simulink library "periodicControllerExp_wCtrlAllocation"  (R2020a)
settings: Solver=VariableStepAuto  StartTime=0.0  StopTime=10.0  RelTol=1e-3
undefined symbols (not defined in the file or in its folder): FLIGHTCONTROLLER, rollAmp, rollFreq, rollKD, rollKP, startControl, tow_speed, vhcl, yawAmp, yawFreq, yawKP
libraries: hiToLoElevationControllerExp x1, ctrlAllocMatrix_cl x1, filteredPIDController_ul x1
settings Model: Creator=jcreed2  LastModifiedBy=jcreed2

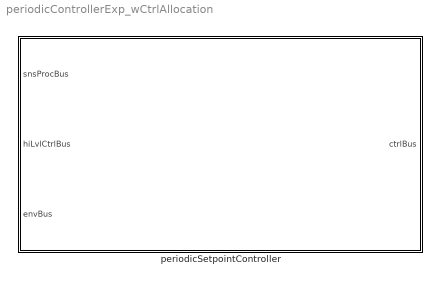
== system periodicControllerExp_wCtrlAllocation ==
  periodicSetpointController : Subsystem  VariantControl=strcmpi(FLIGHTCONTROLLER,'periodicSetpointController')

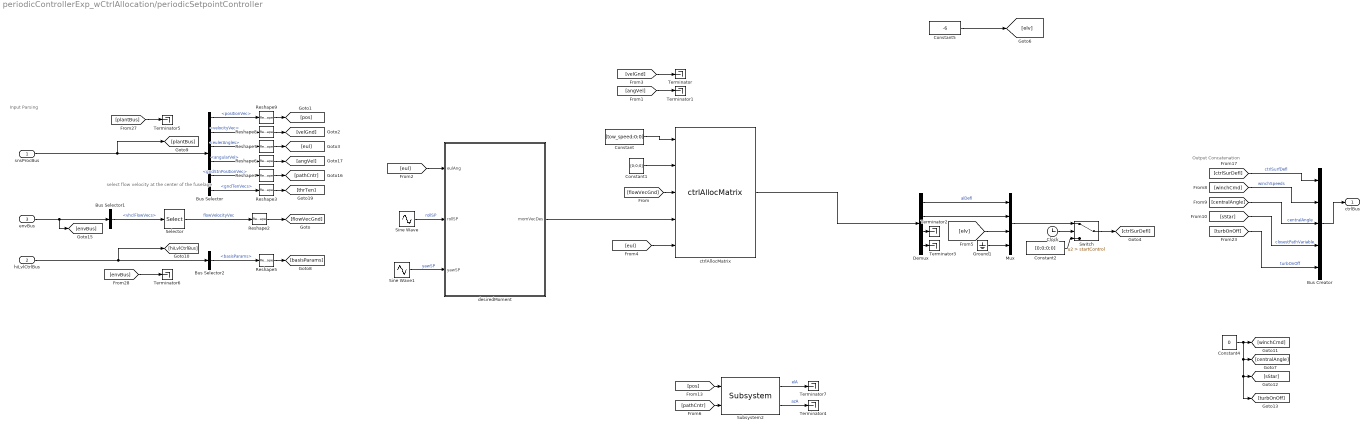
== system periodicControllerExp_wCtrlAllocation/periodicSetpointController ==
  note: select flow velocity at the center of the fuselage
  note: Input Parsing
  note: Output Concatenation
  snsProcBus : Inport  OutDataTypeStr=Bus: sensorsProcessingBus
  hiLvlCtrlBus : Inport  Port=2  OutDataTypeStr=Bus: hiLvlCtrlBus
  envBus : Inport  Port=3  OutDataTypeStr=Bus: envBus
  Bus Creator : BusCreator  Inputs=5  OutDataTypeStr=Bus: fltCtrlBus
      settings: InheritFromInputs=off
  Bus Selector : BusSelector  OutputSignals=positionVec,velocityVec,eulerAngles,angularVel,gndStnPositionVec,gndTenVecs
  Bus Selector1 : BusSelector  OutputSignals=vhclFlowVecs
  Bus Selector2 : BusSelector  OutputSignals=basisParams
  Clock : Clock
  Constant : Constant  Value=[tow_speed;0;0]
  Constant1 : Constant  Value=[0;0;0]
  Constant2 : Constant  Value=[0;0;0;0]
  Constant4 : Constant  Value=0
  Constant5 : Constant  Value=-6
  Demux : Demux
  Ground1 : Ground
  Mux : Mux
  Reshape{1..3,5..9} (8 alike) : Reshape  OutputDimensionality=Column vector (2-D)
  Selector : Selector  NumberOfDimensions=2  InputPortWidth=3  IndexOptions=Select all,Index vector (dialog)  Indices=[1 3],5  OutputSizes=1,1
  Sine Wave : Sin  Amplitude=rollAmp  Bias=180  Frequency=rollFreq  SampleTime=0
  Sine Wave1 : Sin  Amplitude=yawAmp  Bias=pi  Frequency=yawFreq  SampleTime=0
  Subsystem2 : hiToLoElevationControllerExp/hiToLoElevationControllerExp/Subsystem  SystemSampleTime=-1  Latency=0  AutoFrameSizeCalculation=off
  Switch : Switch  Criteria=u2 > Threshold  Threshold=startControl  ZeroCross=off
  Terminator{,1..7} (8 alike) : Terminator
  ctrlAllocMatrix : ctrlAllocMatrix_cl/ctrlAllocMatrix  aeroStruct=vhcl.struct('OCT.aeroSurf')  fluidDensity=1000
  desiredMoment : Subsystem  mask{rollKp=rollKP, rollKd=rollKD, rollTau=.02, yawKp=yawKP}
      mask prompts: rollKp "roll kp"; rollKd "roll kd"; rollTau "roll time constant"; yawKp "yaw kp"
  ctrlBus : Outport  OutDataTypeStr=Bus: fltCtrlBus  VectorParamsAs1DForOutWhenUnconnected=off
  wires:
  Sine Wave/1 -> desiredMoment/2(rollSP)  "rollSP"
  [velGnd] -> Terminator/1
  Sine Wave1/1 -> desiredMoment/3(yawSP)  "yawSP"
  [eul] -> ctrlAllocMatrix/5
  [angVel] -> Terminator1/1
  [flowVecGnd] -> ctrlAllocMatrix/3
  [eul] -> desiredMoment/1(eulAng)
  Bus Selector/2 -> Reshape8/1  "<velocityVec>"
  Reshape3/1 -> [thrTen]
  Bus Selector/5 -> Reshape1/1  "<gndStnPositionVec>"
  Bus Selector/1 -> Reshape9/1  "<positionVec>"
  Reshape5/1 -> [basisParams]
  Reshape1/1 -> [pathCntr]
  envBus/1 -> [envBus], Bus Selector1/1
  snsProcBus/1 -> Bus Selector/1, [plantBus]
  hiLvlCtrlBus/1 -> [hiLvlCtrlBus], Bus Selector2/1
  Reshape2/1 -> [flowVecGnd]
  Bus Selector/4 -> Reshape6/1  "<angularVel>"
  Selector/1 -> Reshape2/1  "flowVelocityVec"
  Bus Selector2/1 -> Reshape5/1  "<basisParams>"
  Bus Selector/6 -> Reshape3/1  "<gndTenVecs>"
  [envBus] -> Terminator6/1
  Reshape6/1 -> [angVel]
  Reshape9/1 -> [pos]
  Bus Selector/3 -> Reshape7/1  "<eulerAngles>"
  Bus Selector1/1 -> Selector/1  "<vhclFlowVecs>"
  [plantBus] -> Terminator5/1
  Reshape7/1 -> [eul]
  Reshape8/1 -> [velGnd]
  [ctrlSurDefl] -> Bus Creator/1  "ctrlSurfDefl"
  [centralAngle] -> Bus Creator/3  "centralAngle"
  [turbOnOff] -> Bus Creator/5  "turbOnOff"
  [winchCmd] -> Bus Creator/2  "winchSpeeds"
  [sStar] -> Bus Creator/4  "closestPathVariable"
  Bus Creator/1 -> ctrlBus/1
  Constant4/1 -> [turbOnOff], [sStar], [centralAngle], [winchCmd]
  [elv] -> Mux/3
  desiredMoment/1(momVecDes) -> ctrlAllocMatrix/4
  Constant/1 -> ctrlAllocMatrix/1
  Constant1/1 -> ctrlAllocMatrix/2
  ctrlAllocMatrix/1 -> Demux/1
  Demux/1 -> Mux/1  "alDefl"
  Demux/2 -> Mux/2
  Ground1/1 -> Mux/4
  Constant5/1 -> [elv]
  Demux/3 -> Terminator2/1
  Demux/4 -> Terminator3/1
  Subsystem2/1 -> Terminator7/1  "elA"
  [pathCntr] -> Subsystem2/2
  [pos] -> Subsystem2/1
  Subsystem2/2 -> Terminator4/1  "azA"
  Clock/1 -> Switch/2
  Constant2/1 -> Switch/3
  Switch/1 -> [ctrlSurDefl]
  Mux/1 -> Switch/1

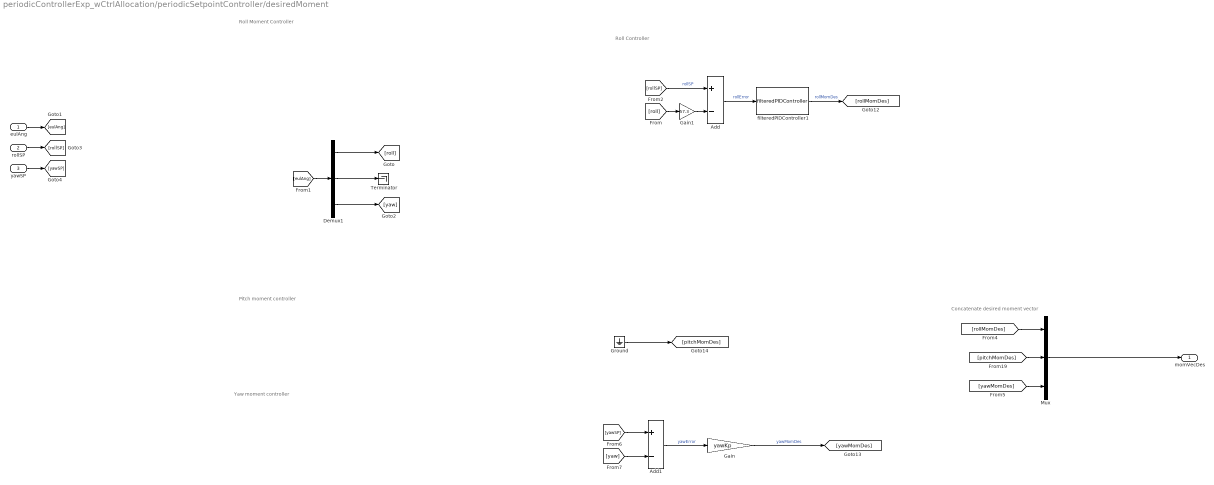
== system periodicControllerExp_wCtrlAllocation/periodicSetpointController/desiredMoment ==
  note: Pitch moment controller
  note: Roll Controller
  note: Yaw moment controller
  note: Roll Moment Controller
  note: Concatenate desired moment vector
  eulAng : Inport
  rollSP : Inport  Port=2
  yawSP : Inport  Port=3
  Add : Sum  Inputs=+-
  Add1 : Sum  Inputs=+-
  Demux1 : Demux  Outputs=3
  Gain : Gain  Gain=yawKp
  Gain1 : Gain  Gain=57.3
  Ground : Ground
  Mux : Mux  Inputs=3
  Terminator : Terminator
  filteredPIDController1 : filteredPIDController_ul/filteredPIDController  kp=rollKp  ki=0  kd=rollKd  Value=rollTau  externalReset=none
  momVecDes : Outport  VectorParamsAs1DForOutWhenUnconnected=off
  wires:
  [pitchMomDes] -> Mux/2
  filteredPIDController1/1 -> [rollMomDes]  "rollMomDes"
  Mux/1 -> momVecDes/1
  [rollMomDes] -> Mux/1
  Ground/1 -> [pitchMomDes]
  [yawMomDes] -> Mux/3
  Add/1 -> filteredPIDController1/1  "rollError"
  [eulAng] -> Demux1/1
  Demux1/2 -> Terminator/1
  Demux1/1 -> [roll]
  Demux1/3 -> [yaw]
  eulAng/1 -> [eulAng]
  [roll] -> Gain1/1
  yawSP/1 -> [yawSP]
  rollSP/1 -> [rollSP]
  [yawSP] -> Add1/1
  [yaw] -> Add1/2
  Add1/1 -> Gain/1  "yawError"
  Gain/1 -> [yawMomDes]  "yawMomDes"
  [rollSP] -> Add/1  "rollSP"
  Gain1/1 -> Add/2
